simulink model "mLossMaps"  (R2021b)
settings: Solver=VariableStepAuto  StartTime=0.0  StopTime=10.0  RelTol=1e-3
model workspace (MAT data in the model file):
  AdjacencyMat = [0 0 0 0 0 0 0 0 0 0 0 0 ... (15129 elements, 123x123)]
  AmatND = [-2.65077937969e-20 -2.66038954729e-20 -2.67754578621e-20 -2.65078353535e-20 -2.66039370332e-20 -2.677549943e-20 -2.6507849929e-20 -2.660395161e-20 -2.67755140094e-20 -2.63787781554e-20 -2.64749060874e-20 -2.66465404e-20 ... (1633932 elements, 3x3x3x2x2x123x123)]
  BkptsStruct.w = [1000 2000 4000]
  BkptsStruct.fr1 = [1 3 10]
  BkptsStruct.fr2 = [1 2.5 7]
  BkptsStruct.Tin1 = [15 50]
  BkptsStruct.Tin2 = [20 60]
  BmatND = [1e-20 1e-20 1e-20 1e-20 1e-20 1e-20 1e-20 1e-20 1e-20 1e-20 1e-20 1e-20 ... (1633932 elements, 3x3x3x2x2x123x123)]
  CapMat = [1e+20; 2196.70091586; 387.653102799; 193.8265514; 1962.34710525; 387.653102799; 193.8265514; 1962.34710525; 1266.59353814; 268.053957132; 416.539515956; 175.715078; 577.243160678; 310.101557898; 23.9530731873; 15.4990473565; 47.9061463746; 30.998094713; 86.96376; 1.05359370745; 1.05359370745; 1.05359370745; 1.05359370745; 1.05359370745; 1.05359370745; 0.351197902483; 0.351197902483; 450.202206395; 54.9511679003; 54.9511679003; 247.389926005; 247.389926005; 75.306462; 75.306462; 1.05359370745; 1.05359370745; 1e+20; 1e+20; 0; 0; 0; 0; 429.469897824; 0; 0; 0; 0; 429.469897824; 0; 0; 0; 0; 0; 0; 424.408023296; 268.053957132; 0; 0; 0; 0; 0; 322.102423368; 0; 0; 0; 0; 0; 322.102423368; 0; 0; 0; 0; 0; 318.306017472; 268.053957132; 2196.70091586; 1266.59353814; 268.053957132; 416.539515956; 175.715078; 577.243160678; 310.101557898; 86.96376; 0.351197902483; 0.351197902483; 450.202206395; 0; 0; 0; 0; 0; 424.408023296; 268.053957132; 0; 0; 0; 0; 318.306017472; 268.053957132; 2196.70091586; 1266.59353814; 268.053957132; 416.539515956; 175.715078; 577.243160678; 310.101557898; 86.96376; 0.351197902483; 0.351197902483; 450.202206395; 0; 0; 0; 0; 0; 424.408023296; 268.053957132; 0; 0; 0; 0; 318.306017472; 268.053957132]
  CoolantArrayIdxs = [20; 21; 22; 23; 24; 25; 26; 27; 35; 36; 37; 84; 85; 108; 109; 19; 38; 83; 107]
  Friction_Loss_Mat = [0 0 0 0 0 0 0 0 0 0 0 0 ... (2340 elements, 39x60)]
  InletCoolIdxs = [37; 38]
  Iron_Loss_Rotor_Back_Iron_Mat = [0.0117705351991 0.0191199073272 0.027445349141 0.0367468606406 0.0470244418259 0.058278092697 0.0705078132537 0.0837136034962 0.0978954634244 0.113053393038 0.129187392338 0.146297461323 ... (2340 elements, 39x60)]
  Iron_Loss_Rotor_Pole_Mat = [1.45649756865 2.73308858082 4.37524107823 6.38295506088 8.75623052876 11.4950674819 14.5994659202 18.0694258438 21.9049472526 26.1060301467 30.672674526 35.6048803905 ... (2340 elements, 39x60)]
  Iron_Loss_Rotor_Tooth_Mat = [0 0 0 0 0 0 0 0 0 0 0 0 ... (2340 elements, 39x60)]
  Iron_Loss_Stator_Back_Iron_Mat = [38.5419456951 60.2019391448 83.4546129961 108.299967249 134.738001903 162.768716959 192.392112416 223.608188275 256.416944535 290.818381197 326.81249826 364.399295724 ... (2340 elements, 39x60)]
  Iron_Loss_Stator_Tooth_Mat = [42.0610884508 66.4921951458 93.1903434872 122.155533475 153.387765109 186.88703839 222.653353317 260.686709891 300.98710811 343.554547977 388.389029489 435.490552649 ... (2340 elements, 39x60)]
  LossDistrForEachType = [0 0 0 0 0 0 0 0 0 0 0 0 ... (1968 elements, 16x123)]
  Magnet_Loss_Mat = [0.0995193918038 0.21922656949 0.383923994091 0.592930489194 0.845728039973 1.14189916514 1.4810945944 1.863014369 2.28739582812 2.7540054971 3.26263335352 3.81308862512 ... (2340 elements, 39x60)]
  OutletCoolIdxs = [20; 107]
  ResMatND = [0 0 0 0 0 0 0 0 0 0 0 0 ... (1633932 elements, 3x3x3x2x2x123x123)]
  Rotor_Cage_Loss_Mat = [0 0 0 0 0 0 0 0 0 0 0 0 ... (2340 elements, 39x60)]
  ShaftTorqueVec = [-287.262157301 -272.268610731 -257.275064161 -242.281517591 -227.287971021 -212.294424451 -197.300877881 -182.307331311 -167.31378474 -152.32023817 -137.3266916 -122.33314503 -107.33959846 -92.34605189 -77.35250532 -62.3589587499 -47.3654121798 -32.3718656097 -17.3783190396 -2.38477246955 12.6087741005 27.6023206706 42.5958672407 57.5894138108 72.5829603809 87.576506951 102.570053521 117.563600091 132.557146661 147.550693231 162.544239801 177.537786371 192.531332942 207.524879512 222.518426082 237.511972652 252.505519222 267.499065792 282.492612362]
  SpeedVec = [500 661.016949153 822.033898305 983.050847458 1144.06779661 1305.08474576 1466.10169492 1627.11864407 1788.13559322 1949.15254237 2110.16949153 2271.18644068 2432.20338983 2593.22033898 2754.23728814 2915.25423729 3076.27118644 3237.28813559 3398.30508475 3559.3220339 3720.33898305 3881.3559322 4042.37288136 4203.38983051 4364.40677966 4525.42372881 4686.44067797 4847.45762712 5008.47457627 5169.49152542 5330.50847458 5491.52542373 5652.54237288 5813.55932203 5974.57627119 6135.59322034 6296.61016949 6457.62711864 6618.6440678 6779.66101695 6940.6779661 7101.69491525 7262.71186441 7423.72881356 7584.74576271 7745.76271186 7906.77966102 8067.79661017 8228.81355932 8389.83050847 8550.84745763 8711.86440678 8872.88135593 9033.89830508 9194.91525424 9355.93220339 9516.94915254 9677.96610169 9838.98305085 10000]
  StatorCopperTempCoefResistivity = 0.00393
  Stator_Copper_Loss_Mat = [3925.33912093 3510.19452231 3089.33767218 2711.80000483 2370.99356953 2062.06508217 1781.35176729 1526.02799256 1293.87708125 1083.15658499 892.54525431 720.809889245 ... (2340 elements, 39x60)]
  Stray_Load_Loss_Mat = [0 0 0 0 0 0 0 0 0 0 0 0 ... (2340 elements, 39x60)]
  Tgiven = 20
  TnodesInit = [25; 25; 25; 25; 25; 25; 25; 25; 25; 25; 25; 25; 25; 25; 25; 25; 25; 25; 25; 25; 25; 25; 25; 25; 25; 25; 25; 25; 25; 25; 25; 25; 25; 25; 25; 25; 25; 25; 25; 25; 25; 25; 25; 25; 25; 25; 25; 25; 25; 25; 25; 25; 25; 25; 25; 25; 25; 25; 25; 25; 25; 25; 25; 25; 25; 25; 25; 25; 25; 25; 25; 25; 25; 25; 25; 25; 25; 25; 25; 25; 25; 25; 25; 25; 25; 25; 25; 25; 25; 25; 25; 25; 25; 25; 25; 25; 25; 25; 25; 25; 25; 25; 25; 25; 25; 25; 25; 25; 25; 25; 25; 25; 25; 25; 25; 25; 25; 25; 25; 25; 25; 25; 25]
  Windage_Loss_Mat = [0 0 0 0 0 0 0 0 0 0 0 0 ... (2340 elements, 39x60)]
  speedVal = 2000
  torqueVal = 20
libraries: mcadROM_lib x1
settings Model: Creator=agonzale  LastModifiedBy=agonzale

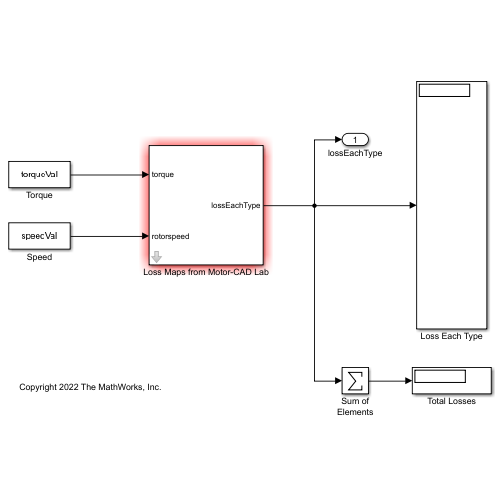
[thumbnail: Simulink's stored preview of the top-level diagram]
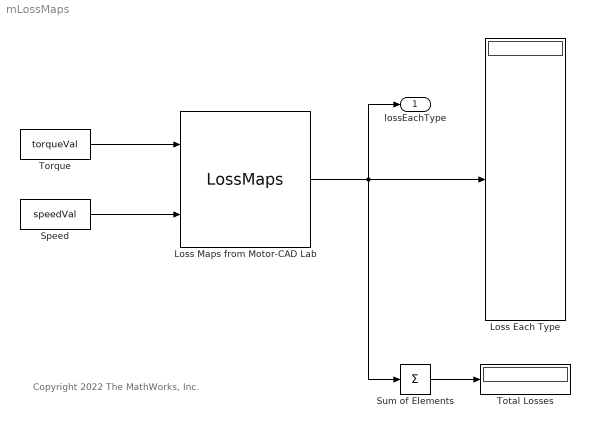
== system mLossMaps ==
  note: Copyright 2022 The MathWorks, Inc.
  Loss Each Type : Display
  Loss Maps from Motor-CAD Lab : mcadROM_lib/LossMaps  ShaftTorqueVec=ShaftTorqueVec  SpeedVec=SpeedVec  Stator_Copper_Loss_Mat=Stator_Copper_Loss_Mat  Rotor_Cage_Loss_Mat=Rotor_Cage_Loss_Mat  Iron_Loss_Stator_Back_Iron_Mat=Iron_Loss_Stator_Back_Iron_Mat  Iron_Loss_Stator_Tooth_Mat=Iron_Loss_Stator_Tooth_Mat  Stray_Loss_Stator_Iron_Proportion=Stray_Loss_Stator_Iron_Proportion  Stray_Load_Loss_Mat=Stray_Load_Loss_Mat  Magnet_Loss_Mat=Magnet_Loss_Mat  Iron_Loss_Rotor_Pole_Mat=Iron_Loss_Rotor_Pole_Mat  Iron_Loss_Rotor_Back_Iron_Mat=Iron_Loss_Rotor_Back_Iron_Mat  Iron_Loss_Rotor_Tooth_Mat=Iron_Loss_Rotor_Tooth_Mat  Friction_Loss_Mat=Friction_Loss_Mat  Windage_Loss_Mat=Windage_Loss_Mat
  Speed : Constant  Value=speedVal
  Sum of Elements : Sum  Inputs=+
  Torque : Constant  Value=torqueVal
  Total Losses : Display
  lossEachType : Outport
  wires:
  Torque/1 -> Loss Maps from Motor-CAD Lab/1
  Speed/1 -> Loss Maps from Motor-CAD Lab/2
  Loss Maps from Motor-CAD Lab/1 -> Sum of Elements/1, lossEachType/1, Loss Each Type/1
  Sum of Elements/1 -> Total Losses/1
